simulink model "RCAM_model_Measurements"  (R2022b)
settings: Solver=VariableStepAuto  StartTime=0.0  StopTime=TF  RelTol=1e-3
values from neighbouring files (symbols this model uses):
  U0 = [0 ... (first row only)    [RCAM_model_initialConditions.m]    (also in designPIL.m)
  X0 = [100 ... (first row only)    [RCAM_model_initialConditions.m]    (also in designPIL.m = [85)
  XYZ0 = [0;0;0]    [RCAM_model_initialConditions.m]    (also in designPIL.m)
undefined symbols (not defined in the file or in its folder): RCAM_model
libraries: sharedtransform x1
settings Model: Creator=bendr  LastModifiedBy=bendr

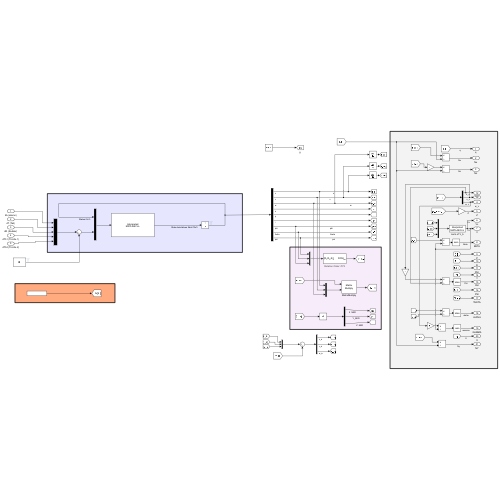
[thumbnail: Simulink's stored preview of the top-level diagram]
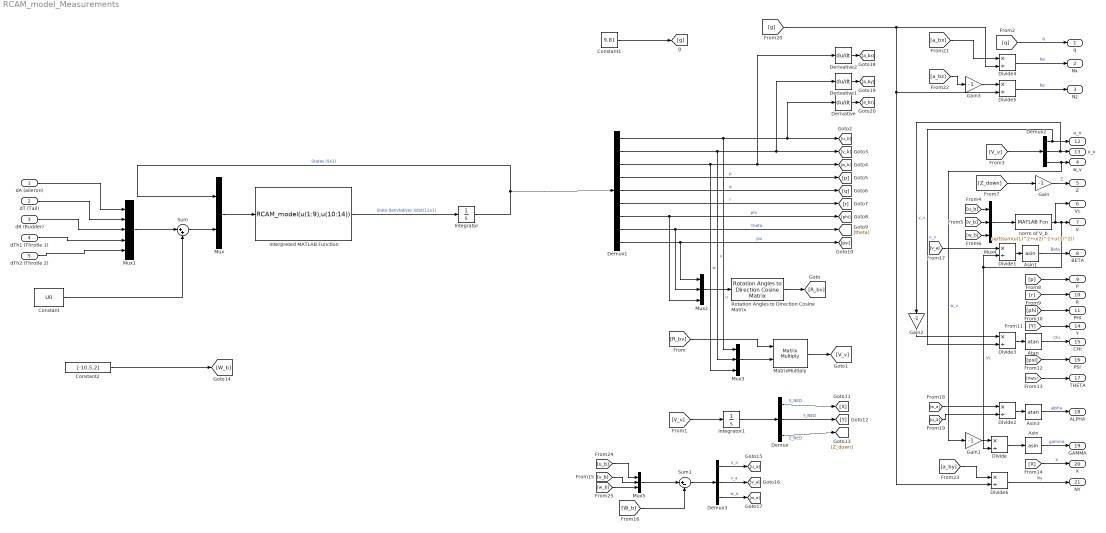
== system RCAM_model_Measurements ==
  dA (aileron) : Inport
  dT (Tail) : Inport  Port=2
  dR (Rudder) : Inport  Port=3
  dTh1 (Throtle 1) : Inport  Port=4
  dTh2 (Throtle 2) : Inport  Port=5
  Asin : Trigonometry  Operator=asin
  Asin1 : Trigonometry  Operator=asin
  Asin3 : Trigonometry  Operator=atan
  Atan : Trigonometry  Operator=atan
  Constant : Constant  Value=U0
  Constant1 : Constant  Value=9.81
  Constant2 : Constant  Value=[-10,5,2]
  Demux : Demux  Outputs=3
  Demux1 : Demux  Outputs=9
  Demux2 : Demux  Outputs=3
  Demux3 : Demux  Outputs=3
  Derivative : Derivative
  Derivative1 : Derivative
  Derivative2 : Derivative
  Divide{,1..6} (7 alike) : Product  Inputs=*/
  Gain{,1..3} (4 alike) : Gain  Gain=-1
  Integrator : Integrator  InitialCondition=X0
  Integrator1 : Integrator  InitialCondition=XYZ0
  Interpreted MATLAB Function : MATLABFcn  MATLABFcn=RCAM_model(u(1:9),u(10:14))
  MatrixMultiply : Product  Multiplication=Matrix(*)
  Mux : Mux  Inputs=2
  Mux1 : Mux  Inputs=5
  Mux{2..5} (4 alike) : Mux  Inputs=3
  Rotation Angles to Direction Cosine Matrix : sharedtransform/Rotation Angles to Direction Cosine Matrix  rotationOrder=ZYX  aMode=aMode
  Sum : Sum  Inputs=|++
  Sum1 : Sum  Inputs=|+-
  norm of V_b : MATLABFcn  MATLABFcn=sqrt(sum(u(1)^2+u(2)^2+u(3)^2))
  q : Outport
  Nx : Outport  Port=2
  Nz : Outport  Port=3
  w_v : Outport  Port=4
  Z : Outport  Port=5
  Vc : Outport  Port=6
  V : Outport  Port=7
  BETA : Outport  Port=8
  P : Outport  Port=9
  R : Outport  Port=10
  PHI : Outport  Port=11
  u_v : Outport  Port=12
  v_v : Outport  Port=13
  Y : Outport  Port=14
  CHI : Outport  Port=15
  PSI : Outport  Port=16
  THETA : Outport  Port=17
  ALPHA : Outport  Port=18
  GAMMA : Outport  Port=19
  X : Outport  Port=20
  NY : Outport  Port=21
  wires:
  Interpreted MATLAB Function/1 -> Integrator/1  "State derivtatives Xdot(12x1)"
  dA (aileron)/1 -> Mux1/1
  Constant/1 -> Sum/2
  Mux/1 -> Interpreted MATLAB Function/1
  dT (Tail)/1 -> Mux1/2
  dR (Rudder)/1 -> Mux1/3
  dTh2 (Throtle 2)/1 -> Mux1/5
  dTh1 (Throtle 1)/1 -> Mux1/4
  Sum/1 -> Mux/2
  Mux1/1 -> Sum/1
  Integrator/1 -> Mux/1, Demux1/1  "States (9x1)"
  Asin1/1 -> BETA/1  "Beta"
  Constant1/1 -> [g]
  Derivative1/1 -> [a_by]
  Atan/1 -> CHI/1  "Chi"
  [a_by] -> Divide6/1
  Gain3/1 -> Divide5/1
  [Y] -> Y/1
  Demux3/1 -> [u_a]  "u_a"
  Mux5/1 -> Sum1/1
  [W_b] -> Sum1/2
  [psi] -> PSI/1
  [Z_down] -> Gain/1
  Demux2/2 -> v_v/1, Gain2/1  "v_v"
  Demux1/5 -> [q]  "q"
  [w_b] -> Mux4/3
  [a_bx] -> Divide4/1
  Demux1/8 -> Mux2/2, [theta]  "theta"
  Rotation Angles to Direction Cosine Matrix/1 -> [R_bv]
  [v_a] -> Divide1/1
  Demux/1 -> [X]  "X_NED"
  [v_b] -> Mux5/2
  Sum1/1 -> Demux3/1
  [phi] -> PHI/1
  Demux1/2 -> Mux3/2, Derivative1/1, [v_b]  "v"
  Demux/3 -> [Z_down]  "Z_NED"
  [V_v] -> Integrator1/1
  [w_b] -> Mux5/3
  [a_bz] -> Gain3/1
  [u_b] -> Mux4/1
  Demux1/4 -> [p]  "p"
  Divide3/1 -> Atan/1
  Mux2/1 -> Rotation Angles to Direction Cosine Matrix/1
  Demux/2 -> [Y]  "Y_NED"
  [u_b] -> Mux5/1
  [r] -> R/1
  [R_bv] -> MatrixMultiply/1
  Mux4/1 -> norm of V_b/1
  Demux1/9 -> Mux2/1, [psi]  "psi"
  Derivative/1 -> [a_bz]
  Demux1/7 -> Mux2/3, [phi]  "phi"
  Divide4/1 -> Nx/1  "Nx"
  Demux1/3 -> Mux3/3, Derivative2/1, [w_b]  "w"
  Divide6/1 -> NY/1  "Ny"
  [g] -> Divide4/2, Divide6/2, Divide5/2
  [theta] -> THETA/1
  Asin/1 -> GAMMA/1  "gamma"
  [q] -> q/1  "q"
  [V_v] -> Demux2/1
  [w_a] -> Divide2/1
  Demux2/3 -> Gain1/1, w_v/1  "w_v"
  norm of V_b/1 -> Vc/1, Divide/2, Divide1/2, V/1  "Vc"
  Gain2/1 -> Divide3/1
  [v_b] -> Mux4/2
  Integrator1/1 -> Demux/1
  [p] -> P/1
  Demux3/3 -> [w_a]  "w_a"
  Derivative2/1 -> [a_bx]
  MatrixMultiply/1 -> [V_v]
  [X] -> X/1  "X"
  Gain1/1 -> Divide/1
  [u_a] -> Divide2/2
  Mux3/1 -> MatrixMultiply/2
  Divide/1 -> Asin/1
  Gain/1 -> Z/1  "Z"
  Divide2/1 -> Asin3/1
  Demux1/1 -> Mux3/1, Derivative/1, [u_b]  "u"
  Demux3/2 -> [v_a]  "v_a"
  Divide1/1 -> Asin1/1
  Demux1/6 -> [r]  "r"
  Demux2/1 -> Divide3/2, u_v/1  "u_v"
  Asin3/1 -> ALPHA/1  "alpha"
  Divide5/1 -> Nz/1  "Nz"
  Constant2/1 -> [W_b]
